simulink library "PooliirAccelRmdl"  (R2022b)
settings: Solver=VariableStepAuto  StartTime=0.0  StopTime=10.0  RelTol=1e-3
undefined symbols (not defined in the file or in its folder): frameSize, maxNumStages, numChannels, numStages, Row, sosCoefficients
libraries: TuneVar x4, TOP x2, AudioStats x1, FeaturePath x1, ITC x1
settings Model: Creator=sd49596  LastModifiedBy=jk1043656
settings SolverCC: AlgebraicLoopSolver=TrustRegion
settings DebuggingCC: UnconnectedInputMsg=warning  UnconnectedOutputMsg=warning  UnconnectedLineMsg=warning  SFMachineParentedDataDiag=warning  ArithmeticOperatorsInVariantConditions=warning
settings ModelReferenceCC: EnableRefExpFcnMdlSchedulingChecks=on
settings SFSimCC: CustomCodeUndefinedFunction=UseInterfaceOnly
settings RTWCC: DLArmComputeVersion=19.05

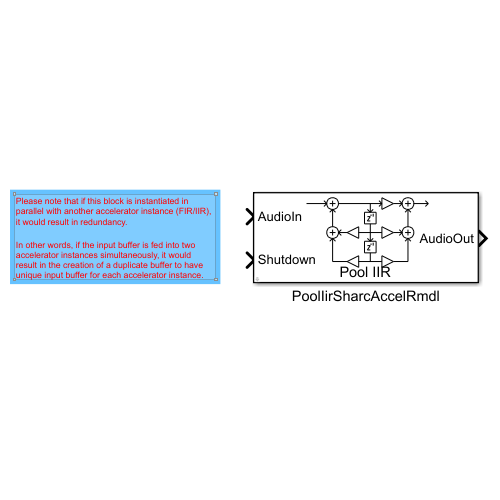
[thumbnail: Simulink's stored preview of the top-level diagram]
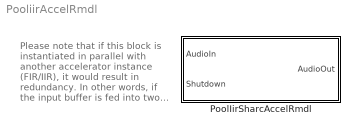
== system PooliirAccelRmdl ==
  note: Please note that if this block is instantiated in parallel with another accelerator instance (FIR/IIR), it would result in redundancy.
      |
      | In other words, if the input buffer is fed into two accelerator instances simultaneously, it would result in the creation of a duplicate buffer to have unique input buffer for each accelerator instance.
  PoolIirSharcAccelRmdl : Subsystem  mask(Bose Pool IIR){variantSelect=Core, maxNumStages=maxNumStages, numStages=numStages, sosCoefficients=sosCoefficients, frameSize=frameSize, numChannels=numChannels, FeatureName=FeatureName}
      mask prompts: variantSelect "Implementation"; maxNumStages "Maximum number of stages"; numStages "Number of stages per channel"; sosCoefficients "Coefficient pool"; frameSize "Frame size"; numChannels "Number of channels"; FeatureName "Filter name/purpose"
      mask help:
      | Pool IIR is a configurable multi-channel IIR filter that supports one or more channels.  Different filter coefficients and number of stages (biquads) can be used for each channel filter.  The Pool IIR model supports two different implementations, selectable from the model mask:
      |
      | (i)  Core: IIR filters executing on core
      | (ii) Accel: IIR filters executing on IIR hardware accelerator, offloading MIPS usage from core
      |
      | NOTE: The Pool IIR codeWorkMemory buffer should always be mapped to L1 memory or core MIPS usage will increase.
      |
      | For more information, please see 'Help'.
      mask init:
      | % Create alias for code work memory buffer for each instance of model
      | PooliirAccelMask(gcbh);
      | 
      | % There are three implementation types:
      | % Type    Value  Description
      | % CORE    1      Optimized assembly running on core
      | % ACCEL   2      Computing offloaded to accelerator peripheral
      | % GENERIC 3      Generic implementation for other targets without CRL
      | 
      | PostOverlayRequired = ( variantSelect == 2 );
      | if variantSelect == 1
      |     % State memory used for core implementation
      |     codeWorkMemorySize = 2*maxNumStages;
      |     
      | elseif variantSelect == 2
      |     % Accelerator CRL code work memory size is equal to:
      |     %             sizeof(iirAccelWorkMemory_t) + variableDataSize;
      |     % with variable data size dependent on number channels and 
      |     % frame size.  NOTE: this must be updated to match the CRL code
      |     % if any changes are made to the accelWorkMemory_t structure.
      |     cacheLineLen = 64;  % ADI GUL size in bytes
      |     variableDataSize = TargetCacheRoundUpSize( ...
      |                               (64 + numChannels * (64 + frameSize * 4)), ...
      |                               1, ...
      |                               cacheLineLen); % bytes
      |     codeWorkMemorySize = 64 + variableDataSize; % bytes
      |     codeWorkMemorySize = codeWorkMemorySize / 4; % words (single)
      |     
      | else
      |     % This is not used if there is no CRL
      |     codeWorkMemorySize = 1;
      | end
      mask Help:
      | <b>Input signals: </b>
      | AudioIn: input channels [frame size x number of channels]
      | 
      | <b>Output signals: </b>
      | AudioOut: output channels [frame size x number of channels]
      | 
      | <b>Mask parameters: </b>
      | Implementation: Core/Accel
      | Maximum number of stages [scalar]
      | Number of stages per channel [1 x number of channels]
      | Coefficient pool [total number of stages x 6]
      | Frame size [scalar]
      | Number of channels [scalar]
      | Filter name/purpose
      mask TypeOptions variantSelect: Core | Accel
      mask Callback variantSelect:
      | % Get the mask parameter value
      | maskStr = get_param(gcb,'variantSelect');
      | 
      | % Check the value of 'variantSelect'
      | if (strcmp(maskStr,"Core"))
      |     % Turn the visibility of 'frameSize' and 'numChannels' OFF
      |     set_param(gcb,'MaskVisibilities',{'on';'on';'on';'on';'off';'off';'on'});
      | else
      |     % "Accel": Set the visibility of all parameters to ON
      |     set_param(gcb,'MaskVisibilities',{'on';'on';'on';'on';'on';'on';'on'});
      | end
      mask TypeOptions numStages: Tune Variable1/MaskValue
      mask TypeOptions sosCoefficients: Tune Variable/MaskValue
      mask TypeOptions FeatureName: FeaturePath/FeatureName
      mask Display:
      | [path,w,h] = IconIIR_Mask();
      | 
      | % work in pixels since the icon does not scale
      | pos = get(gcbh,'position');
      | bw = pos(3) - pos(1);
      | bh = pos(4) - pos(2);
      | 
      | % Draw centered icon
      | xAdj = bw/2 - w/2;
      | yAdj = bh/2 - h/2 + 4;
      | for i=1:length(path)
      | %     patch(path(i).x+xAdj, path(i).y+yAdj, path(i).rgb);
      |     plot(path(i).x+xAdj, path(i).y+yAdj);
      | end
      | 
      | % Anchor the corners of the coordinate system
      | patch(0,0,[1 1 1]);
      | patch(bw,bh,[1 1 1]);
      | 
      | % Display some text
      | text(bw/2, 1,'Pool IIR', ...
      |     'horizontalAlignment','center', ...
      |     'VerticalAlignment','bottom');

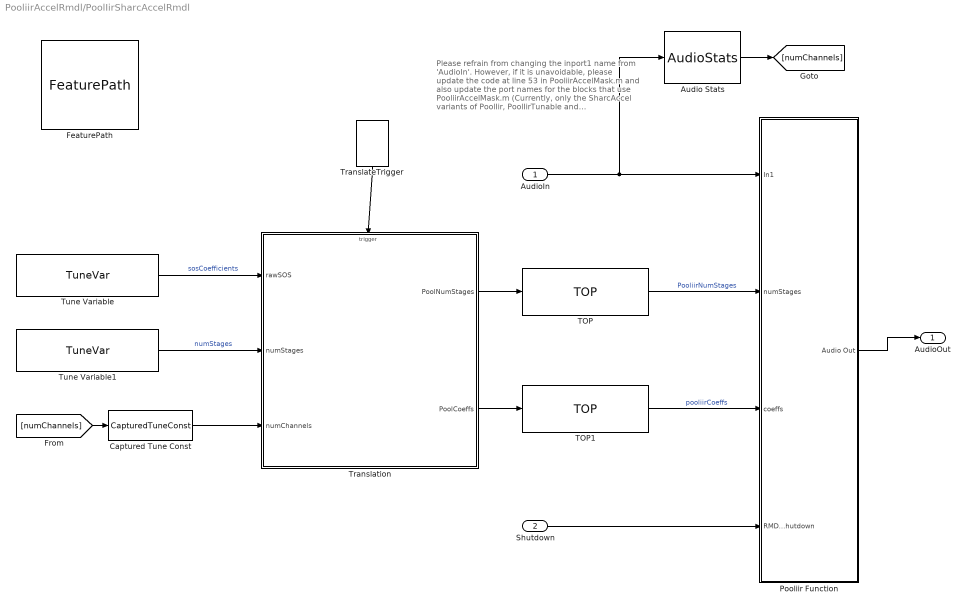
== system PooliirAccelRmdl/PoolIirSharcAccelRmdl ==
  note: Please refrain from changing the inport1 name from 'AudioIn'. However, if it is unavoidable, please update the code at line 53 in PooliirAccelMask.m and also update the port names for the blocks that use PooliirAccelMask.m (Currently, only the SharcAccel variants of PoolIir, PoolIirTunable and PooliirAccelRmdl block use that.)
  AudioIn : Inport
  Shutdown : Inport  Port=2
  Audio Stats : AudioStats/AudioStats  DoSampleRate=off  TypeSampleRate=Inherit: auto  DoCallRate=off  TypeCallRate=Inherit: auto  DoFrameSize=off  TypeFrameSize=Inherit: auto  DoChannelCount=on  TypeChannelCount=Inherit: auto  DoTaskRateFactor=off  TypeTaskRateFactor=Inherit: auto  MacroNameRoot=AUDIO  MacroNameRootEval='AUDIO'  IsMacroNameEval=off  MacroSampleRate=off  MacroCallRate=off  MacroFrameSize=off  MacroChannelCount=off  MacroTaskRateFactor=off  MacroTaskId=off  ValidateSampleRate=off  ValueSampleRate=[]  ValidateCallRate=off  ValueCallRate=[]  ValidateFrameSize=off  ValueFrameSize=[]  ValidateChannelCount=off  ValueChannelCount=[]  ValidateTaskRateFactor=off  ValueTaskRateFactor=[]
      settings: SourceProductName=Bose Talaria
  Captured Tune Const : TuneVar/CapturedTuneConst  TriggerInit=[-640 382 -540 418]  Role=Automatic
      settings: SourceProductName=Bose Talaria
  FeaturePath : FeaturePath/FeaturePath  FeatureName=FeatureName  IsGroup=off  GroupNumber=-1  IsModule=off  TriggerInit=[-720 -61 -605 46]
      settings: SourceProductName=Bose Talaria
  Pooliir Function : Subsystem
  TOP : TOP/TOP  TriggerInit=[-145 212 5 268]  TopName=PooliirNumStages  DataType=uint32  BankNumber=0  PreOverlay=false  PostOverlay=PostOverlayRequired  Role=Automatic
      settings: SourceProductName=Bose Talaria
  TOP1 : TOP/TOP  TriggerInit=[-145 352 5 408]  TopName=pooliirCoeffs  DataType=single  BankNumber=0  PreOverlay=false  PostOverlay=PostOverlayRequired  Role=Automatic
      settings: SourceProductName=Bose Talaria
  TranslateTrigger : TuneVar/TranslateTrigger  TriggerInit=[-344 35 -306 90]
      settings: SourceProductName=Bose Talaria
  Translation : MATLAB Function  TreatAsAtomicUnit=on
  Tune Variable : TuneVar/TuneVar  TuneName=sosCoefficients  SpecifyMaxSize=on  VariableDim=1 (Row)  MaxSize=[maxNumStages 6]  TunabilityNumber=1  MinValue=[]  MaxValue=[]  TriggerInit=[-750 195 -580 245]  MaskValue=sosCoefficients
      settings: SourceProductName=Bose Talaria
  Tune Variable1 : TuneVar/TuneVar  TuneName=numStages  SpecifyMaxSize=off  VariableDim=1 (Row)  MaxSize=[1 1]  TunabilityNumber=1  MinValue=[]  MaxValue=[]  TriggerInit=[-750 285 -580 335]  MaskValue=numStages
      settings: SourceProductName=Bose Talaria
  AudioOut : Outport  VectorParamsAs1DForOutWhenUnconnected=off
  wires:
  AudioIn/1 -> Audio Stats/1, Pooliir Function/1(In1)
  TOP/1 -> Pooliir Function/2(numStages)  "PooliirNumStages"
  TOP1/1 -> Pooliir Function/3(coeffs)  "pooliirCoeffs"
  Pooliir Function/1(Audio Out) -> AudioOut/1
  TranslateTrigger/1 -> Translation/Trigger
  Tune Variable/1 -> Translation/1(rawSOS)  "sosCoefficients"
  Translation/2(PoolCoeffs) -> TOP1/1
  Translation/1(PoolNumStages) -> TOP/1
  Tune Variable1/1 -> Translation/2(numStages)  "numStages"
  Audio Stats/1 -> [numChannels]
  [numChannels] -> Captured Tune Const/1
  Captured Tune Const/1 -> Translation/3(numChannels)
  Shutdown/1 -> Pooliir Function/4(RMDL Shutdown)

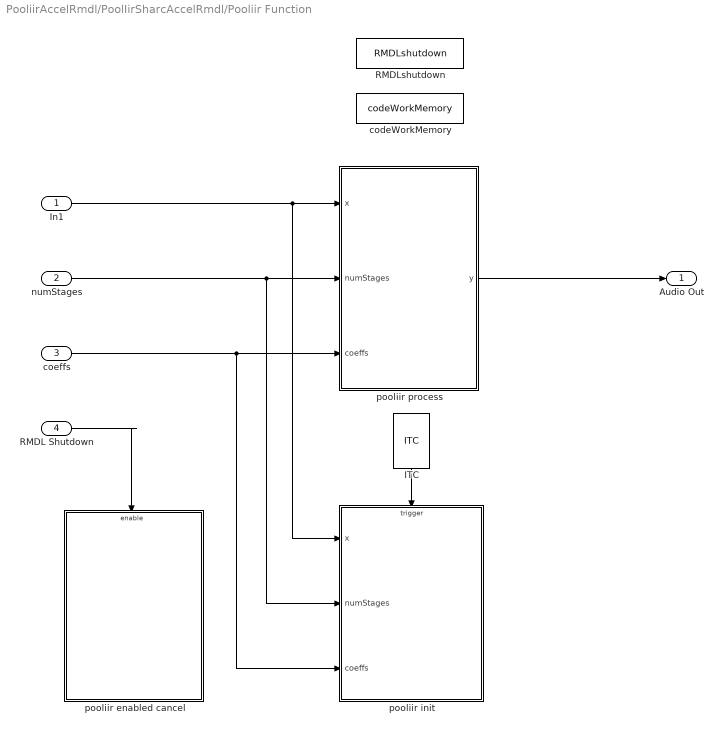
== system PooliirAccelRmdl/PoolIirSharcAccelRmdl/Pooliir Function ==
  In1 : Inport
  numStages : Inport  Port=2
  coeffs : Inport  Port=3
  RMDL Shutdown : Inport  Port=4
  ITC : ITC/ITC
      settings: SourceProductName=Bose Talaria
  RMDLshutdown : DataStoreMemory  DataStoreName=RMDLshutdown  WriteAfterWriteMsg=warning  ShowAdditionalParam=off  OutDataTypeStr=uint32  Dimensions=[1,1]
      settings: LockScale=on
  codeWorkMemory : DataStoreMemory  DataStoreName=codeWorkMemory  WriteAfterWriteMsg=warning  InitialValue=zeros(1,codeWorkMemorySize)  EmbeddedSignalClassName=Blocklib.Signal  ShowAdditionalParam=off  OutDataTypeStr=single
  pooliir enabled cancel : Subsystem  TreatAsAtomicUnit=on
  pooliir init : MATLAB Function  TreatAsAtomicUnit=on  RTWFcnName=foo
  pooliir process : MATLAB Function  TreatAsAtomicUnit=on
  Audio Out : Outport  VectorParamsAs1DForOutWhenUnconnected=off
  wires:
  ITC/1 -> pooliir init/Trigger
  pooliir process/1(y) -> Audio Out/1
  In1/1 -> pooliir init/1(x), pooliir process/1(x)
  numStages/1 -> pooliir process/2(numStages), pooliir init/2(numStages)
  coeffs/1 -> pooliir process/3(coeffs), pooliir init/3(coeffs)
  RMDL Shutdown/1 -> pooliir enabled cancel/Enable

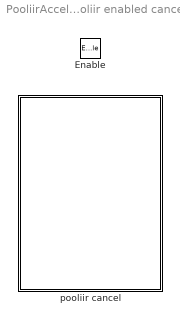
== system PooliirAccelRmdl/PoolIirSharcAccelRmdl/Pooliir Function/pooliir enabled cancel ==
  Enable : EnablePort
  pooliir cancel : MATLAB Function  TreatAsAtomicUnit=on

== matlab function PooliirAccelRmdl/PoolIirSharcAccelRmdl/Pooliir Function/pooliir init ==
  data: x input; numStages input; coeffs input; codeWorkMemory data_store_memory; variantSelect parameter; RMDLshutdown data_store_memory
  events: trigger input FUNCTION_CALL_EVENT
function pooliir_init(x, numStages, coeffs, variantSelect)
% Process function for Pooliir
%
% Parameters:
%   x:              input channels [frame size x number of inputs]
%   numStages:      coefficient sets [total filter lengths x 1]
%   coeffs:         array of filter lengths [number of filters x 1]
%
% Global parameters:
%   codeWorkMemory: working memory set up during roommode reset/init CRL
%                   function call [codeWorkMemorySize x 1]
%   RMDLshutdown: Flag to indicate RMDL is in progress [1 x 1]

% Extract configuration information from inputs
[frame_size, num_channels] = size(x);

% Initialize variables
global codeWorkMemory;
global RMDLshutdown;

% Get the work memory size
workMemorySize = numel(codeWorkMemory);

% Set correct data types
frame_size = uint32(frame_size);
num_channels = uint32(num_channels);
workMemorySize = uint32(workMemorySize);

% There are two implementation types:
% Type   Value   Description
% CORE   1       Optimized assembly running on core
% ACCEL  2       Computing offloaded to accelerator peripheral

% NOTE: Core variant does not need any custom initialization

if (variantSelect == 2)
    y = pooliirAccelInit(x, frame_size, num_channels, numStages, coeffs, ...
                         codeWorkMemory, workMemorySize);

    % NOTE: The CRL mechanism requires an output for the function call,
    % and appears to be optimized out if that return value isn't used. 
    % This is a dummy operation to make sure CRL ends up in generated code
    codeWorkMemory(1) = y; 
end

% Set flag to indicate initialization has completed and step functions can
% start running.
RMDLshutdown = uint32(1);

end


function y = pooliirAccelInit(x, frame_size, num_channels, numStages, coeffs, ...
                              workMemory, workMemorySize)
% If target == codegen, error out if no CRL found
coder.replace('-errorifnoreplacement');

% No init simulation code, but need to do something to ensure CRL does not
% get optimized out
y = workMemory(1) + 1;

end

== matlab function PooliirAccelRmdl/PoolIirSharcAccelRmdl/Pooliir Function/pooliir process ==
  data: x input; numStages input; y output; coeffs input; variantSelect parameter; codeWorkMemory data_store_memory; RMDLshutdown data_store_memory
function y = pooliir_process(x, numStages, coeffs, variantSelect)
% Process function for Pooliir
%
% Parameters:
%   x:              input channels [frame size x number of inputs]
%   numStages:      coefficient sets [total filter lengths x 1]
%   coeffs:         array of filter lengths [number of filters x 1]
%
% Global parameters:
%   codeWorkMemory: working memory set up during roommode reset/init CRL
%                   function call [codeWorkMemorySize x 1]
%   RMDLshutdown: Flag to indicate RMDL is in progress [1 x 1]

% Extract configuration information from inputs
[frame_size, num_channels] = size(x);

% Initialize variables
global codeWorkMemory;
global RMDLshutdown;

% Do not call the step processing functions if RMDL shutdown is in
% progress
if (RMDLshutdown == 0)
    y = zeros(frame_size, num_channels, 'single');
    return;
end
        
% Set correct data types
frame_size = uint32(frame_size);
num_channels = uint32(num_channels);

% There are two implementation types:
% Type   Value   Description
% CORE   1       Optimized assembly running on core
% ACCEL  2       Computing offloaded to accelerator peripheral
if (variantSelect == 1)
    % Core selection
    % Call wrapper function for simulation and code generation
    y = pooliirCore(x, frame_size, num_channels, numStages, coeffs, codeWorkMemory);
elseif (variantSelect == 2)
    % Accelerator selection
    if(coder.target('MATLAB') || coder.target('Sfun'))
        % Accelerator simulation
        y = pooliirAccel(x, frame_size, num_channels, numStages, coeffs);
    else
        % Accelerator code generation
        y = iir_accelerator_process(x, codeWorkMemory);
    end
else
    error('Invalid implementation type');
end

end

function y = iir_accelerator_process(x, workMemory)
% If target == codegen, error out if no CRL found
coder.replace('-errorifnoreplacement');

[frameSize, numChannels]  = size(x);
y = zeros(frameSize, numChannels, 'single');
end

== matlab function PooliirAccelRmdl/PoolIirSharcAccelRmdl/Translation ==
  data: rawSOS input; numStages input; numChannels input; PoolNumStages output; PoolCoeffs output; maxNumStages parameter; variantSelect parameter
  events: trigger input FUNCTION_CALL_EVENT
function [PoolNumStages, PoolCoeffs] = pooliirTranslation(rawSOS, numStages, numChannels, maxNumStages, variantSelect)
% Translation from raw SOS for pool SOS

% Some build time sanity size checking before calling the translation
if numel(numStages.Value) ~= numChannels
    error('Size of num stages has to match number of input channels')
end
if rawSOS.Size(2) ~= 6
    error ('Coefficient pool matrix must have 6 columns')
end

% There are two implementation types:
% Type   Value   Description
% CORE   1       Optimized assembly running on core
% ACCEL  2       Computing offloaded to accelerator peripheral
if (variantSelect == 1)
    [PoolNumStages, PoolCoeffs] = pooliirTranslationFcn(rawSOS, numStages, maxNumStages);
elseif (variantSelect == 2)
    [PoolNumStages, PoolCoeffs] = pooliirAccelTranslationFcn(rawSOS, numStages, maxNumStages);
else
    TranslateError('Invalid implementation type');
end

end

== matlab function PooliirAccelRmdl/PoolIirSharcAccelRmdl/Pooliir Function/pooliir enabled cancel/pooliir cancel ==
  data: variantSelect parameter; codeWorkMemory data_store_memory; RMDLshutdown data_store_memory
function pooliir_cancel(variantSelect)

% IIR accelerator function stops step/process function from running on each
% frame and cancels IIR accelerator task if currently active.
% 
% Parameters:
%   None
%
% Global parameters:
%   codeWorkMemory: Working memory set up during roommode reset/init CRL
%                   function call [1 x codeWorkMemorySize]
%   RMDLshutdown: Flag to indicate RMDL is in progress [1 x 1] 

global codeWorkMemory;
global RMDLshutdown;

% Clear flag to indicate RMDL shutdown has started. Note that this flag
% will be set after RMDL and initialization have completed.
RMDLshutdown = uint32(0);

% There are two implementation types:
% Type   Value   Description
% CORE   1       Optimized assembly running on core
% ACCEL  2       Computing offloaded to accelerator peripheral
if(~coder.target('MATLAB') && ~coder.target('Sfun')) 
    % Code Generation
    if (variantSelect == 2)
        y = pooliirAccelCancel(codeWorkMemory);

        % NOTE: The CRL mechanism requires an output for the function call,
        % and appears to be optimized out if that return value isn't used. 
        % This is a dummy operation to make sure CRL ends up in generated code
        codeWorkMemory(1) = y;
    end
end

end


% IIR accelerator CRL cancel function conceptual specification
function y = pooliirAccelCancel(workMemory)
% If target == codegen, error out if no CRL found
coder.replace('-errorifnoreplacement');

% No cancel simulation code, but need to do something to ensure CRL does not
% get optimized out
y = uint32(workMemory(1) + 1);

end
